simulink subsystem "rms_detector_sub"  (R2023a)
settings: Solver=VariableStepAuto  StartTime=0.0  StopTime=10.0  RelTol=1e-3
libraries: dspstat3 x1
settings Model: Creator=ElvisJu  LastModifiedBy=ElvisJu

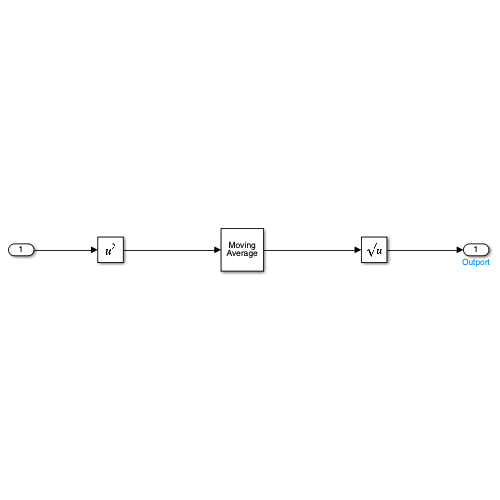
[thumbnail: Simulink's stored preview of the top-level diagram]
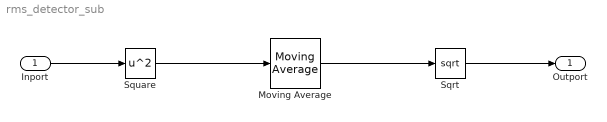
== system rms_detector_sub ==
  Inport : Inport
  Moving Average : dspstat3/Moving Average  Method=Sliding window  ForgettingFactorPort=off  SpecifyWindowLength=on  WindowLength=500  OverlapLength=3  AllowArbitraryInputLength=off  ForgettingFactor=0.9  SimulateUsing=Code generation
  Sqrt : Sqrt
  Square : Math  Operator=square
  Outport : Outport
  wires:
  Sqrt/1 -> Outport/1
  Moving Average/1 -> Sqrt/1
  Square/1 -> Moving Average/1
  Inport/1 -> Square/1
